simulink model "Lab1_1"  (Simulink 7.3)
settings: Solver=ode3  StartTime=0.0  StopTime=8  FixedStep=0.001  RelTol=1e-3
undefined symbols (not defined in the file or in its folder): MultiQ, PCI, Quanser
libraries: rtwinlib x2
settings Model: Creator=Mehatronicki Sustavi  LastModifiedBy=Mehatronicki Sustavi  SimulationMode=external  ExtModeTrigDuration=1000000
settings HardwareCC: ProdIntDivRoundTo=Zero  ProdEndianess=LittleEndian  ProdHWDeviceType=Generic->32-bit x86 compatible
settings RTWCC: SystemTargetFile=rtwin.tlc  TemplateMakefile=rtwin.tmf  Description=Real-Time Windows Target  ProcessScript=rtwin_make_rtw_hook  RTWCompilerOptimization=On
settings CodeAppCC: MaxIdLength=95
settings RTWinTargetCC: TargetFunctionLibrary=ANSI_C  PortableWordSizes=off

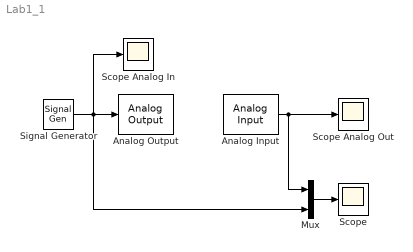
== system Lab1_1 ==
  Analog Input : rtwinlib/Analog Input  SampleTime=0.001  DrvName=Quanser/MultiQ-PCI  DrvAddress=4294967295  DrvOptions=zeros(1,0)  Channels=1  RangeMode=1  VoltRange=1  DataType=1
      settings: AttributesFormatString=Quanser\nMultiQ-PCI [auto]
  Analog Output : rtwinlib/Analog Output  SampleTime=0.001  DrvName=Quanser/MultiQ-PCI  DrvAddress=4294967295  DrvOptions=zeros(1,0)  Channels=1  RangeMode=1  VoltRange=1  InitialValue=[]  FinalValue=[]
      settings: AttributesFormatString=Quanser\nMultiQ-PCI [auto]
  Mux : Mux  Inputs=2
  Scope : Scope
      settings: SaveName=SawInOut_16Hz  DataFormat=Array
  Scope Analog In : Scope
      settings: SaveName=SawAnalogIn_16Hz  DataFormat=Array
  Scope Analog Out : Scope
      settings: SaveName=SawAnalogOut_16Hz  DataFormat=Array
  Signal Generator : SignalGenerator  WaveForm=sawtooth  Amplitude=3  Frequency=16
  wires:
  Signal Generator/1 -> Analog Output/1, Scope Analog In/1, Mux/2
  Analog Input/1 -> Scope Analog Out/1, Mux/1
  Mux/1 -> Scope/1
